simulink model "ZControlado"  (R2018b)
settings: Solver=VariableStepAuto  StartTime=0.0  StopTime=ttotal  RelTol=1e-3
values from neighbouring files (symbols this model uses):
  tmuestra = 0.05    [ABCIncremental.m]    (also in ABCLQR.m)
  Yr = 0.05    [ABCIncremental.m]    (also in ABCLQR.m = 0.1)
undefined symbols (not defined in the file or in its folder): A, B, C, ControlDiscretoBAB
settings Model: Creator=pablo  LastModifiedBy=pablo

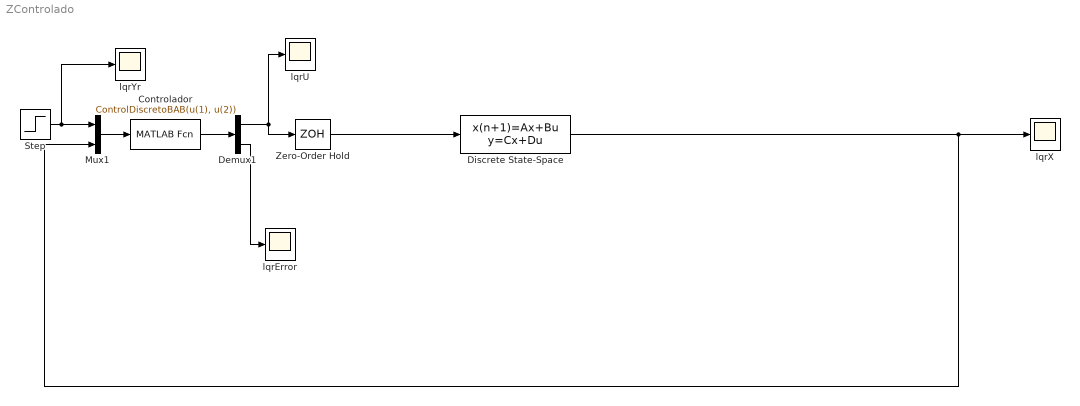
== system ZControlado ==
  Controlador : MATLABFcn  MATLABFcn=ControlDiscretoBAB(u(1), u(2))  OutputDimensions=2
  Demux1 : Demux  Outputs=2
  Discrete State-Space : DiscreteStateSpace  A=A  B=B  C=C  D=0  SampleTime=tmuestra
  Mux1 : Mux  Inputs=2
  Step : Step  After=Yr  SampleTime=tmuestra
  Zero-Order Hold : ZeroOrderHold  SampleTime=tmuestra
  lqrError : Scope
  "lqrU " : Scope
  lqrX : Scope
  "lqrYr " : Scope
  wires:
  Mux1/1 -> Controlador/1
  Step/1 -> "lqrYr "/1, Mux1/1
  Controlador/1 -> Demux1/1
  Demux1/1 -> "lqrU "/1, Zero-Order Hold/1
  Demux1/2 -> lqrError/1
  Zero-Order Hold/1 -> Discrete State-Space/1
  Discrete State-Space/1 -> Mux1/2, lqrX/1
